simulink library "bouyancyCalculator_ul"  (R2018b)
settings: Solver=VariableStepAuto  StartTime=0.0  StopTime=10.0  RelTol=1e-3
values from neighbouring files (symbols this model uses):
  D = sum(normalVecMat'.*relVelGnd',2)    [oceanForceFunct.m]
undefined symbols (not defined in the file or in its folder): gndStn
libraries: vrlib x1, dspmtrx3 x1
settings Model: Creator=jcreed2  LastModifiedBy=jcreed2

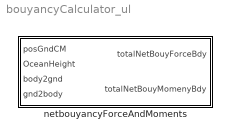
== system bouyancyCalculator_ul ==
  netbouyancyForceAndMoments : Subsystem

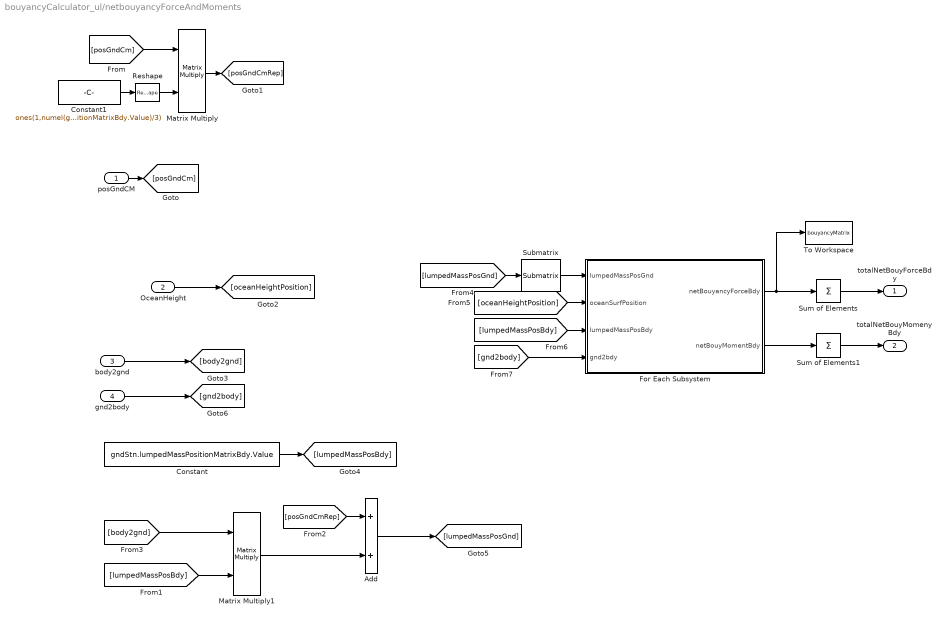
== system bouyancyCalculator_ul/netbouyancyForceAndMoments ==
  posGndCM : Inport
  OceanHeight : Inport  Port=2
  body2gnd : Inport  Port=3
  "gnd2body " : Inport  Port=4
  Add : Sum
  Constant : Constant  Value=gndStn.lumpedMassPositionMatrixBdy.Value
  Constant1 : Constant  Value=ones(1,numel(gndStn.lumpedMassPositionMatrixBdy.Value)/3)
  For Each Subsystem : Subsystem  TreatAsAtomicUnit=on  mask{mR=gndStn.lumpedMassSphereRadius.Value, bouyLM=gndStn.lumpedMassNetBouyancyForce.Value', gravLM=gndStn.gravForcePerLM.Value}
      mask prompts: mR "lumped mass radius"; bouyLM "bouyancy  force per lumped mass"; gravLM "gravity force per lumped mass"
  Matrix Multiply : Product  Multiplication=Matrix(*)
  Matrix Multiply1 : Product  Multiplication=Matrix(*)
  Reshape : Reshape  OutputDimensionality=Row vector (2-D)
  Submatrix : dspmtrx3/Submatrix  RowSpan=One row  RowStartMode=Last  RowStartIndex=1  RowEndMode=Last  RowEndIndex=1  ColSpan=All columns  ColStartMode=First  ColStartIndex=1  ColEndMode=Last  ColEndIndex=1
  Sum of Elements : Sum  Inputs=+  CollapseMode=Specified dimension  CollapseDim=2
  Sum of Elements1 : Sum  Inputs=+  CollapseMode=Specified dimension  CollapseDim=2
  To Workspace : ToWorkspace  VariableName=bouyancyMatrix  SaveFormat=Timeseries  SampleTime=-1
  totalNetBouyForceBdy : Outport
  totalNetBouyMomenyBdy : Outport  Port=2
  wires:
  [lumpedMassPosBdy] -> Matrix Multiply1/2
  Matrix Multiply/1 -> [posGndCmRep]
  For Each Subsystem/2(netBouyMomentBdy) -> Sum of Elements1/1
  [gnd2body] -> For Each Subsystem/4("gnd2bdy ")
  OceanHeight/1 -> [oceanHeightPosition]
  [oceanHeightPosition] -> For Each Subsystem/2(oceanSurfPosition)
  [lumpedMassPosGnd] -> Submatrix/1
  body2gnd/1 -> [body2gnd]
  [body2gnd] -> Matrix Multiply1/1
  Add/1 -> [lumpedMassPosGnd]
  Constant1/1 -> Reshape/1
  [posGndCmRep] -> Add/1
  Sum of Elements1/1 -> totalNetBouyMomenyBdy/1
  [posGndCm] -> Matrix Multiply/1
  Constant/1 -> [lumpedMassPosBdy]
  Matrix Multiply1/1 -> Add/2
  "gnd2body "/1 -> [gnd2body]
  Sum of Elements/1 -> totalNetBouyForceBdy/1
  posGndCM/1 -> [posGndCm]
  For Each Subsystem/1(netBouyancyForceBdy) -> To Workspace/1, Sum of Elements/1
  [lumpedMassPosBdy] -> For Each Subsystem/3(lumpedMassPosBdy)
  Reshape/1 -> Matrix Multiply/2
  Submatrix/1 -> For Each Subsystem/1(lumpedMassPosGnd)

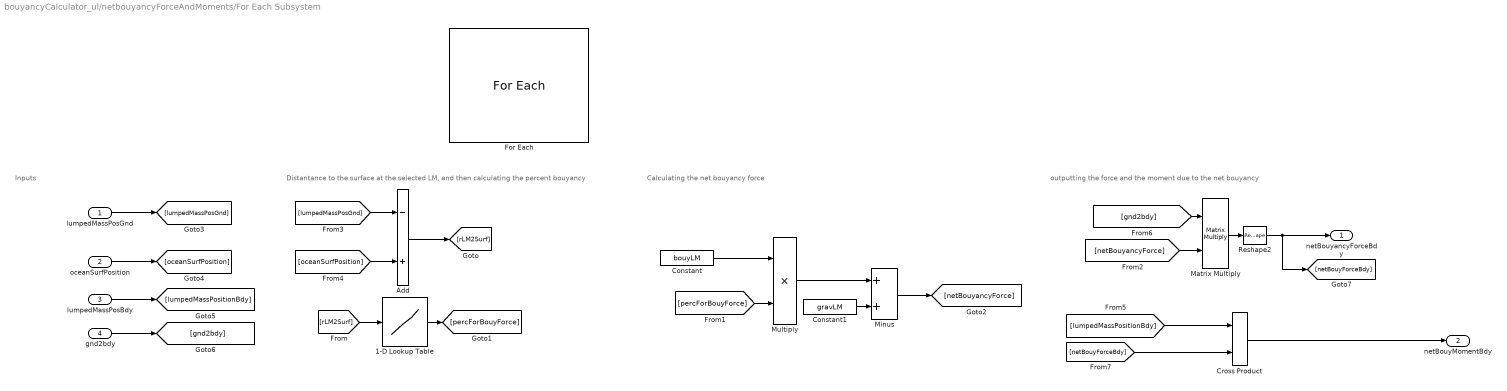
== system bouyancyCalculator_ul/netbouyancyForceAndMoments/For Each Subsystem ==
  note: outputting the force and the moment due to the net bouyancy
  note: Calculating the net bouyancy force
  note: Distantance to the surface at the selected LM, and then calculating the percent bouyancy
  note: Inputs
  lumpedMassPosGnd : Inport  Partition=on  PartitionDimension=2  PartitionWidth=1  PartitionOffset=0
  oceanSurfPosition : Inport  Port=2  Partition=on  PartitionDimension=1  PartitionWidth=1  PartitionOffset=0
  lumpedMassPosBdy : Inport  Port=3  Partition=on  PartitionDimension=2  PartitionWidth=1  PartitionOffset=0
  "gnd2bdy " : Inport  Port=4
  1-D Lookup Table : Lookup_n-D  NumberOfTableDimensions=1  BreakpointsForDimension1=[-mR, .5*-mR, 0, .5*mR, mR]  Table=[0, .25, .5 ,.75,1]  ExtrapMethod=Clip  InternalRulePriority=Speed  RndMeth=Simplest  InputSameDT=on
  Add : Sum  Inputs=-+
  Constant : Constant  Value=bouyLM
  Constant1 : Constant  Value=gravLM
  Cross Product : vrlib/Utilities/Cross Product
      settings: SourceProductBaseCode=VR
  For Each : ForEach  DisableCoverage=on  IndexMode=One-based
  Matrix Multiply : Product  Multiplication=Matrix(*)
  Minus : Sum
  Multiply : Product
  Reshape2 : Reshape  OutputDimensionality=Column vector (2-D)
  netBouyancyForceBdy : Outport  ConcatenationDimension=2
  netBouyMomentBdy : Outport  Port=2  PortDimensions=[3,1]  ConcatenationDimension=2
  wires:
  oceanSurfPosition/1 -> [oceanSurfPosition]
  lumpedMassPosGnd/1 -> [lumpedMassPosGnd]
  Add/1 -> [rLM2Surf]
  [rLM2Surf] -> 1-D Lookup Table/1
  1-D Lookup Table/1 -> [percForBouyForce]
  [percForBouyForce] -> Multiply/2
  Constant/1 -> Multiply/1
  Multiply/1 -> Minus/1
  [netBouyancyForce] -> Matrix Multiply/2
  [lumpedMassPosGnd] -> Add/1
  [oceanSurfPosition] -> Add/2
  [lumpedMassPositionBdy] -> Cross Product/1
  lumpedMassPosBdy/1 -> [lumpedMassPositionBdy]
  "gnd2bdy "/1 -> [gnd2bdy]
  [gnd2bdy] -> Matrix Multiply/1
  Matrix Multiply/1 -> Reshape2/1
  [netBouyForceBdy] -> Cross Product/2
  Cross Product/1 -> netBouyMomentBdy/1
  Reshape2/1 -> [netBouyForceBdy], netBouyancyForceBdy/1
  Constant1/1 -> Minus/2
  Minus/1 -> [netBouyancyForce]
